simulink subsystem "FMC_StateMachineNew_Subsystem"  (R2025a)
settings: Solver=VariableStepAuto  StartTime=0.0  StopTime=10.0  RelTol=1e-3
libraries: simulink x1
settings Model: Creator=MW  LastModifiedBy=MW

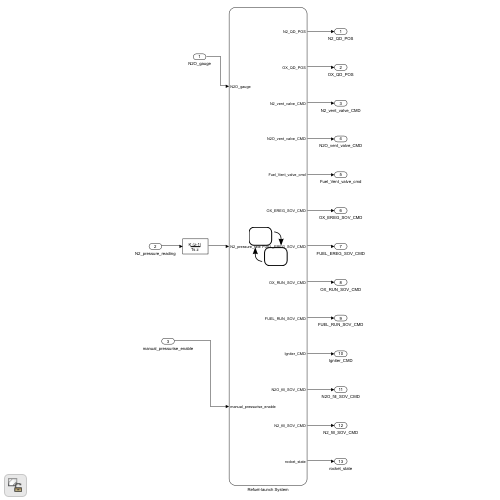
[thumbnail: Simulink's stored preview of the top-level diagram]
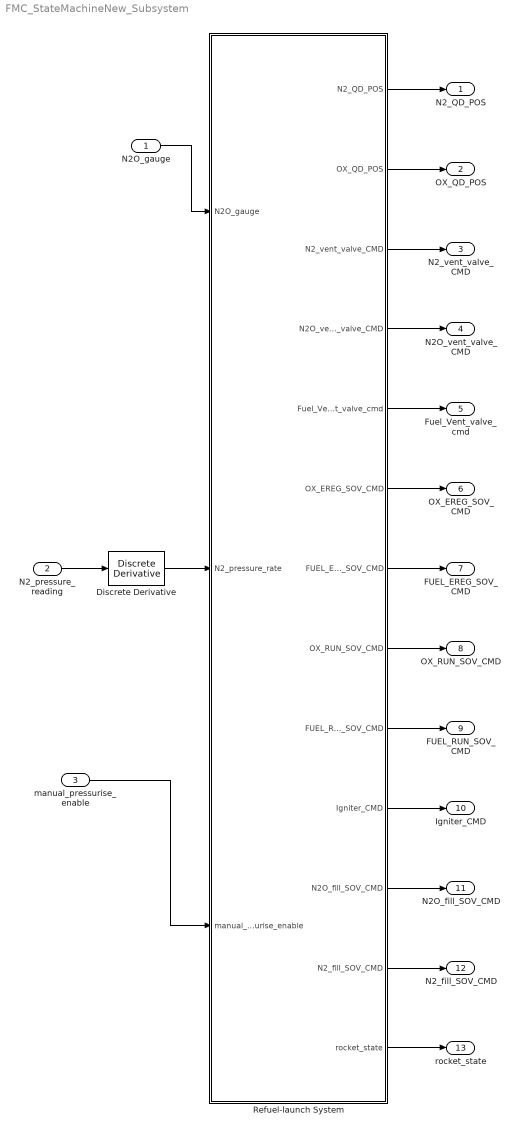
== system FMC_StateMachineNew_Subsystem ==
  N2O_gauge : Inport
  N2_pressure_reading : Inport  Port=2
  manual_pressurise_enable : Inport  Port=3
  Discrete Derivative : simulink/Discrete/Discrete Derivative  gainval=1.0  ICPrevScaledInput=0.0  OutMin=[]  OutMax=[]  OutDataType=fixdt(1, 16)  OutScaling=2^-10  DoSatur=off
  Refuel-launch System : Stateflow chart  TreatAsAtomicUnit=on  SystemSampleTime=0.5
  N2_QD_POS : Outport
  OX_QD_POS : Outport  Port=2
  N2_vent_valve_CMD : Outport  Port=3
  N2O_vent_valve_CMD : Outport  Port=4
  Fuel_Vent_valve_cmd : Outport  Port=5
  OX_EREG_SOV_CMD : Outport  Port=6
  FUEL_EREG_SOV_CMD : Outport  Port=7
  OX_RUN_SOV_CMD : Outport  Port=8
  FUEL_RUN_SOV_CMD : Outport  Port=9
  Igniter_CMD : Outport  Port=10
  N2O_fill_SOV_CMD : Outport  Port=11
  N2_fill_SOV_CMD : Outport  Port=12
  rocket_state : Outport  Port=13
  wires:
  N2O_gauge/1 -> Refuel-launch System/1(N2O_gauge)
  Discrete Derivative/1 -> Refuel-launch System/2(N2_pressure_rate)
  N2_pressure_reading/1 -> Discrete Derivative/1
  manual_pressurise_enable/1 -> Refuel-launch System/3(manual_pressurise_enable)
  Refuel-launch System/1(N2_QD_POS) -> N2_QD_POS/1
  Refuel-launch System/2(OX_QD_POS) -> OX_QD_POS/1
  Refuel-launch System/3(N2_vent_valve_CMD) -> N2_vent_valve_CMD/1
  Refuel-launch System/4(N2O_vent_valve_CMD) -> N2O_vent_valve_CMD/1
  Refuel-launch System/5(Fuel_Vent_valve_cmd) -> Fuel_Vent_valve_cmd/1
  Refuel-launch System/6(OX_EREG_SOV_CMD) -> OX_EREG_SOV_CMD/1
  Refuel-launch System/7(FUEL_EREG_SOV_CMD) -> FUEL_EREG_SOV_CMD/1
  Refuel-launch System/8(OX_RUN_SOV_CMD) -> OX_RUN_SOV_CMD/1
  Refuel-launch System/9(FUEL_RUN_SOV_CMD) -> FUEL_RUN_SOV_CMD/1
  Refuel-launch System/10(Igniter_CMD) -> Igniter_CMD/1
  Refuel-launch System/11(N2O_fill_SOV_CMD) -> N2O_fill_SOV_CMD/1
  Refuel-launch System/12(N2_fill_SOV_CMD) -> N2_fill_SOV_CMD/1
  Refuel-launch System/13(rocket_state) -> rocket_state/1

== stateflow chart FMC_StateMachineNew_Subsystem/Refuel-launch System ==
  state IDLE
    en:
    rocket_state = 0;
    OX_QD_POS = 0;
    N2_QD_POS = 0;
    N2O_vent_valve_CMD = 0;
    Fuel_Vent_valve_cmd = 0;
    N2O_fill_SOV_CMD = 0;
    N2_fill_SOV_CMD = 0;
    OX_RUN_SOV_CMD = 0;
    FUEL_RUN_SOV_CMD = 0;
    Igniter_CMD = 0;
    Fuel_Vent_valve_cmd = 0;
    FUEL_EREG_SOV_CMD = 0;
  state N2O_refueling
    en:
    rocket_state = 1;
    N2O_vent_valve_CMD = 1;
    OX_QD_POS = 1;
    N2O_fill_SOV_CMD = 1;
  state N2O_refueling_complete
    en:
    rocket_state = 2;
    OX_QD_POS = 0;
    N2O_fill_SOV_CMD = 0;
    N2O_vent_valve_CMD = 0;
  state N2_refueling
    en:
    N2_QD_POS = 1;
    rocket_state = 3;
    N2_fill_SOV_CMD = 1;
  state check_progress
    en:
  state N2_refueling_complete
    en:
    N2_QD_POS = 0;
    rocket_state = 4;
    N2_fill_SOV_CMD = 0;
  state Refuel_complete
    en:
    rocket_state = 5;
  state Manual_Pressurisation_WAIT
    en:
    rocket_state = 6;
  state Ignition_precondition
    en:
    rocket_state = 7;
    OX_EREG_SOV_CMD = 1;
    FUEL_EREG_SOV_CMD = 1;
  state Launch
    en:
    rocket_state = 8;
    OX_RUN_SOV_CMD = 1;
    FUEL_RUN_SOV_CMD = 1;
    Igniter_CMD = 1;
  state MECO
    en:
    rocket_state = 9;
    OX_EREG_SOV_CMD = 0;
    OX_RUN_SOV_CMD = 0;
    FUEL_RUN_SOV_CMD = 0;
  state Start_vent
    en:
    rocket_state = 10;
    Fuel_Vent_valve_cmd = 1;
    N2_vent_valve_CMD = 1;
  state Vent_complete
    en:
    rocket_state = 11;
    Fuel_Vent_valve_cmd = 0;
    N2_vent_valve_CMD = 0;
  (default) -> IDLE
  IDLE -> N2O_refueling
  N2O_refueling -> N2O_refueling_complete : [N2O_gauge >= dipstick_gauge_start]
  N2O_refueling_complete -> N2_refueling : after(60, sec)
  N2_refueling -> check_progress : after(60, sec)
  check_progress -> N2_refueling_complete : [N2_pressure_rate<0.01]
  N2_refueling_complete -> Refuel_complete
  Refuel_complete -> Manual_Pressurisation_WAIT : after(200, sec)
  Manual_Pressurisation_WAIT -> Ignition_precondition : [manual_pressurise_enable == 1]
  Ignition_precondition -> Launch : after(10, sec)
  Launch -> MECO : after(2.7, sec)
  MECO -> Start_vent : after(1, sec)
  Start_vent -> Vent_complete : after(5, sec)
  data: N2_QD_POS output; OX_QD_POS output; N2_vent_valve_CMD output; N2O_vent_valve_CMD output; N2O_gauge input; N2_pressure_rate input; Fuel_Vent_valve_cmd output; OX_EREG_SOV_CMD output; FUEL_EREG_SOV_CMD output; OX_RUN_SOV_CMD output; FUEL_RUN_SOV_CMD output; Igniter_CMD output; N2O_fill_SOV_CMD output; N2_fill_SOV_CMD output; rocket_state output; manual_pressurise_enable input; dipstick_gauge_start parameter
